simulink model "Ond_MLI_1"  (R2020a)
settings: Solver=VariableStepAuto  StartTime=0.0  StopTime=1  FixedStep=0.0001  RelTol=1e-3  EnableMultiTasking=on
InitFcn:
  | E=150;
  | V=220;
  | fs=50;
  | A=1;
  | 
  | Teta_0=0;
  | Cr=0;
  | Rr=3.805;
  | J=0.031;
  | f=0;
  | p=2;
  | Rs=4.85;
  | M=0.258;
  | Ls=0.274;
  | Lr=0.274;
  | R=[Rs 0 0 0;0 Rs 0 0;0 0 Rs 0;0 0 0 Rs];
  | L=[Ls 0 M 0;0 Ls 0 M;M 0 Lr 0;0 M 0 Lr];
  | A1=[0 -Ls 0 -M;Ls 0 M 0;0 0 0 0;0 0 0 0];
  | A2=[0 0 0 0;0 0 0 0;0 -M 0 -Lr;M 0 Lr 0];
undefined symbols (not defined in the file or in its folder): Vp
libraries: powerlib x21, simulink x2, powerlib_meascontrol x2
settings Model: SimulationMode=accelerator  Creator=SINA  LastModifiedBy=ABO-CHIFA
settings DataIOCC: ReturnWorkspaceOutputs=off
settings OptimizationCC: LifeSpan=inf
settings DebuggingCC: SFUnexpectedBacktrackingDiag=warning  SFNoUnconditionalDefaultTransitionDiag=warning  ArithmeticOperatorsInVariantConditions=warning
settings SFSimCC: SimUseLocalCustomCode=off  CustomCodeUndefinedFunction=UseInterfaceOnly
settings RTWCC: RTWUseLocalCustomCode=off
settings CodeAppCC: StateflowObjectComments=on
settings GRTTargetCC: TargetLangStandard=C89/C90 (ANSI)
settings ConfigComp: CovMetricSettings=dw  CovHtmlReporting=on  CovSaveCumulativeToWorkspaceVar=on  CovSaveSingleToWorkspaceVar=on  CovExternalEMLEnable=off
settings SimscapeCC: SimscapeNormalizeSystem=off

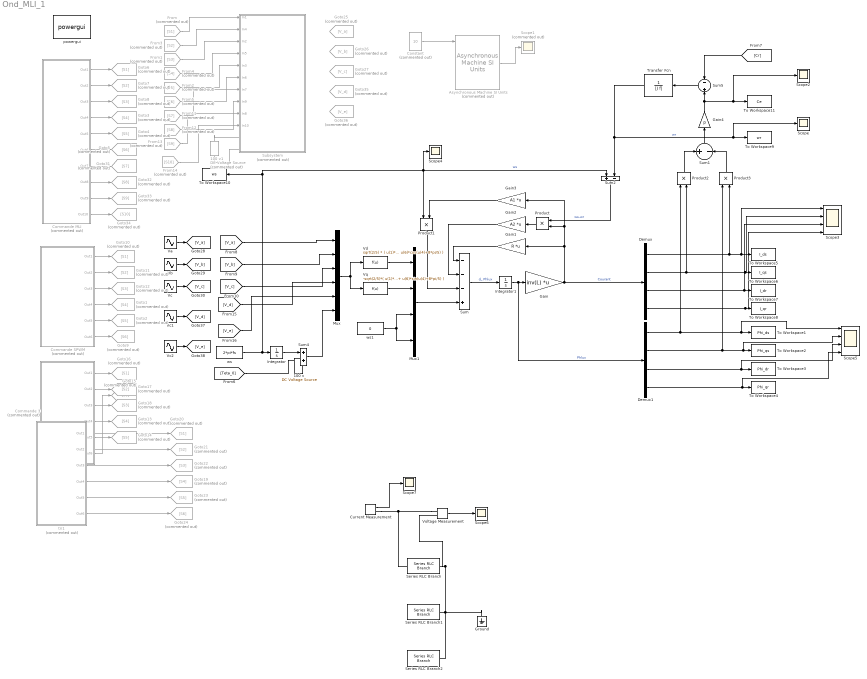
== system Ond_MLI_1 ==
  100 v : powerlib/Electrical Sources/DC Voltage Source  Amplitude=E  Measurements=Voltage
  100 v1 : powerlib/Electrical Sources/DC Voltage Source  Commented=on  Amplitude=E  Measurements=Voltage
  Asynchronous Machine SI Units : powerlib/Machines/Asynchronous Machine SI Units  Commented=on  RotorType=Squirrel-cage  PresetModel="15:  5.4 HP (4KW)   400 V  50Hz 1430 RPM"  MechanicalLoad=Torque Tm  ShowDetailedParameters=on  ReferenceFrame=Rotor  Units=SI  MeasurementBus=off  NominalParameters=[4000 400 50]  Stator=[1.405 0.005839]  Rotor=[1.395 0.005839]  Cage1=[0.4155 0.002066]  Cage2=[0.4168 0.0003495]  Lm=0.1722  Mechanical=[0.0131 0.002985 2]  PolePairs=2  InitialConditions=[1 0 0 0 0 0 0 0]  SimulateSaturation=off  Saturation=[14.03593122, 27.81365428, 53.79336849, 72.68890987, 97.98006896, 148.6815601, 215.7428561, 302.9841135, 428.7778367 ; 230, 322, 414, 460, 506, 552, 598, 644, 690]  LoadFlowParameters=1492000  TsPowergui=0  TsBlock=-1  IterativeModel=Trapezoidal non iterative  IterativeDiscreteModel=Trapezoidal non iterative  Pmec=1.492e+006
  "Commande 3 " : Subsystem  Commented=on
  "Commande MLI " : Subsystem  Commented=on
  "Commande SPWM " : Subsystem  Commented=on
  Constant : Constant  Commented=on  Value=10
  Current Measurement : powerlib/Measurements/Current Measurement  PhasorSimulation=off  OutputType=Complex  PSBequivalent=0
  Demux : Demux
  Demux1 : Demux
  From : From  Commented=on  GotoTag=S1
  From1 : From  Commented=on  GotoTag=S3
  From11 : From  Commented=on  GotoTag=S7
  From12 : From  Commented=on  GotoTag=S8
  From13 : From  Commented=on  GotoTag=S9
  From14 : From  Commented=on  GotoTag=S10
  From2 : From  Commented=on  GotoTag=S5
  From3 : From  Commented=on  GotoTag=S2
  From4 : From  Commented=on  GotoTag=S4
  From5 : From  Commented=on  GotoTag=S6
  Gain : Gain  Gain=inv(L)  Multiplication=Matrix(K*u)
  Gain1 : Gain  Gain=R  Multiplication=Matrix(K*u)
  Gain2 : Gain  Gain=A2  Multiplication=Matrix(K*u)
  Gain3 : Gain  Gain=A1  Multiplication=Matrix(K*u)
  Gain4 : Gain  Gain=p
  Goto{1,3,13,19} (4 alike) : Goto  Commented=on  GotoTag=S4
  Goto{6,10,16,20} (4 alike) : Goto  Commented=on  GotoTag=S1
  Goto{7,11,17,21} (4 alike) : Goto  Commented=on  GotoTag=S2
  Goto{8,12,18,22} (4 alike) : Goto  Commented=on  GotoTag=S3
  Goto{2,4,14,23} (4 alike) : Goto  Commented=on  GotoTag=S5
  Goto{5,9,15,24} (4 alike) : Goto  Commented=on  GotoTag=S6
  Goto25 : Goto  Commented=on  GotoTag=V_a
  Goto26 : Goto  Commented=on  GotoTag=V_b
  Goto27 : Goto  Commented=on  GotoTag=V_c
  Goto31 : Goto  Commented=on  GotoTag=S7
  Goto32 : Goto  Commented=on  GotoTag=S8
  Goto33 : Goto  Commented=on  GotoTag=S9
  Goto34 : Goto  Commented=on  GotoTag=S10
  Goto35 : Goto  Commented=on  GotoTag=V_d
  Goto36 : Goto  Commented=on  GotoTag=V_e
  Ground : powerlib/Elements/Ground  LConnTagsString=a
  Integrator : Integrator
  Integrator1 : Integrator
  Mux : Mux  Inputs=6
  Mux1 : Mux
  Product{,1..3} (4 alike) : Product
  Scope{,2,4,6..7} (5 alike) : Scope
  Scope1 : Scope  Commented=on
  Scope3 : Scope  NumInputPorts=4
  Scope5 : Scope  NumInputPorts=4
  Series RLC Branch : powerlib/Elements/Series RLC Branch  LConnTagsString=__new0  RConnTagsString=__new0  BranchType=R  Resistance=0.1  Inductance=1e-3  SetiL0=off  InitialCurrent=0  Capacitance=1e-6  Setx0=off  InitialVoltage=0  Measurements=None
  Series RLC Branch1 : powerlib/Elements/Series RLC Branch  LConnTagsString=__new0  RConnTagsString=__new0  BranchType=R  Resistance=0.1  Inductance=1e-3  SetiL0=off  InitialCurrent=0  Capacitance=1e-6  Setx0=off  InitialVoltage=0  Measurements=None
  Series RLC Branch2 : powerlib/Elements/Series RLC Branch  LConnTagsString=__new0  RConnTagsString=__new0  BranchType=R  Resistance=0.1  Inductance=1e-3  SetiL0=off  InitialCurrent=0  Capacitance=1e-6  Setx0=off  InitialVoltage=0  Measurements=None
  Subsystem : Subsystem  Commented=on
  Sum : Sum  Inputs=---+
  Sum1 : Sum  Inputs=+-
  Sum2 : Sum  Inputs=+-
  Sum4 : Sum
  Sum5 : Sum  Inputs=-+
  To Workspace1 : ToWorkspace  VariableName=Phi_ds  SampleTime=-1
  To Workspace10 : ToWorkspace  VariableName=ws  SampleTime=-1
  To Workspace11 : ToWorkspace  VariableName=Ce  SampleTime=-1
  To Workspace2 : ToWorkspace  VariableName=Phi_qs  SampleTime=-1
  To Workspace3 : ToWorkspace  VariableName=Phi_dr  SampleTime=-1
  To Workspace4 : ToWorkspace  VariableName=Phi_qr  SampleTime=-1
  To Workspace5 : ToWorkspace  VariableName=I_ds  SampleTime=-1
  To Workspace6 : ToWorkspace  VariableName=I_qs  SampleTime=-1
  To Workspace7 : ToWorkspace  VariableName=I_dr  SampleTime=-1
  To Workspace8 : ToWorkspace  VariableName=I_qr  SampleTime=-1
  To Workspace9 : ToWorkspace  VariableName=wr  SampleTime=-1
  Transfer Fcn : TransferFcn  Denominator=[J f]
  Va : Sin  Amplitude=V*sqrt(2)  Frequency=2*pi*fs  SampleTime=0
  Vb : Sin  Amplitude=V*sqrt(2)  Frequency=2*pi*fs  Phase=2*pi/5  SampleTime=0
  Vc : Sin  Amplitude=V*sqrt(2)  Frequency=2*pi*fs  Phase=4*pi/5  SampleTime=0
  Vc1 : Sin  Amplitude=V*sqrt(2)  Frequency=2*pi*fs  Phase=6*pi/5  SampleTime=0
  Vc2 : Sin  Amplitude=V*sqrt(2)  Frequency=2*pi*fs  Phase=8*pi/5  SampleTime=0
  Vd : Fcn  Expr="sqrt(2/5) * ( u(1)*cos(u(4))  + u(2)*cos(u(4)+2*pi/5) + u(3)*cos(u(4)+4*pi/5)+ u(5)*cos(u(4)+6*pi/5)+ u(6)*cos(u(4)+8*pi/5) )"
  Voltage Measurement : powerlib/Measurements/Voltage Measurement  PhasorSimulation=off  OutputType=Complex  PSBequivalent=0
  Vq : Fcn  Expr="-sqrt(2/5)*( u(1)*sin(u(4))  + u(2)*sin(u(4)+2*pi/5) + u(3)*sin(u(4)+4*pi/5)+ u(5)*sin(u(4)+6*pi/5)+ u(6)*sin(u(4)+8*pi/5) )"
  powergui : powerlib/powergui  Priority=1  SimulationMode=Discrete  SampleTime=1e-6  frequency=60  Iterations=50  frequencyindice=0  Pbase=100e6  ErrMax=1e-4  UnitsV=kV  UnitsW=MW  buscounter=0  FunctionMessages=off  echomessages=off  EnableUseOfTLC=off  CurrentSourceSwitches=off  DisableSnubberDevices=off  DisableRonSwitches=off  DisableVfSwitches=off  DisplayEquations=off  AutomaticDiscreteSolvers=off  SolverType=Tustin/Backward Euler (TBE)  Interpol=off  ExternalGateDelay=off  methode=off  Ts=10  x0status=blocks  SPID=off  SwTol=0  HookPort=off  NonlinearTolerance=1e-4  nMaxIteration=100  ContinueOnMaxIteration=off  RestoreLinks=warning  ResistiveCurrentMeasurement=off  Frange=[0:2:500]  Ylog=off  Xlog=on  ShowGrid=off  save=off  variable=ZData  structure=0  ZoomFFT=off  StartTime=0.0  cycles=1  DisplayStyle=1  fundamental=60  FreqAxis=off  MaxFrequency=1000  frequencyindicesteady=1  RmsSteady=1  display=off
  "tri1 " : Subsystem  Commented=on
  ws : Constant  Value=2*pi*fs
  ws1 : Constant  Value=0
  wires:
  "Commande MLI "/4(Out4) -> Goto3/1
  "Commande MLI "/5(Out5) -> Goto4/1
  "Commande MLI "/6(Out6) -> Goto5/1
  "Commande MLI "/2(Out2) -> Goto7/1
  "Commande MLI "/1(Out1) -> Goto6/1
  "Commande MLI "/3(Out3) -> Goto8/1
  "Commande SPWM "/1(Out1) -> Goto10/1
  "Commande SPWM "/2(Out2) -> Goto11/1
  "Commande SPWM "/3(Out3) -> Goto12/1
  "Commande SPWM "/4(Out4) -> Goto1/1
  "Commande SPWM "/5(Out5) -> Goto2/1
  "Commande SPWM "/6(Out6) -> Goto9/1
  From/1 -> Subsystem/1(In1)
  From1/1 -> Subsystem/3(In2)
  From2/1 -> Subsystem/5(In3)
  From3/1 -> Subsystem/2(In4)
  From4/1 -> Subsystem/4(In5)
  From5/1 -> Subsystem/6(In6)
  "Commande 3 "/1(Out1) -> Goto16/1
  "Commande 3 "/2(Out2) -> Goto17/1
  "Commande 3 "/3(Out3) -> Goto18/1
  "Commande 3 "/4(Out4) -> Goto13/1
  "Commande 3 "/5(Out5) -> Goto14/1
  "Commande 3 "/6(Out6) -> Goto15/1
  Asynchronous Machine SI Units/1 -> Scope1/1
  Constant/1 -> Asynchronous Machine SI Units/1
  "tri1 "/1(Out1) -> Goto20/1
  "tri1 "/2(Out2) -> Goto21/1
  "tri1 "/3(Out3) -> Goto22/1
  "tri1 "/4(Out4) -> Goto19/1
  "tri1 "/5(Out5) -> Goto23/1
  "tri1 "/6(Out6) -> Goto24/1
  ws/1 -> Sum2/1, Scope4/1, Product1/1, To Workspace10/1, Integrator/1  "ws"
  Mux/1 -> Vd/1, Vq/1
  Vd/1 -> Mux1/1
  Vq/1 -> Mux1/2
  ws1/1 -> Mux1/3, Mux1/4
  Sum/1 -> Integrator1/1  "d_ Phlux"
  Integrator1/1 -> Gain/1, Demux1/1  "Phlux"
  Gain/1 -> Demux/1, Gain3/1, Product/2, Gain1/1  "Courant"
  Product/1 -> Gain2/1
  Gain3/1 -> Product1/2
  Demux1/1 -> Product2/1, Scope5/1, To Workspace1/1
  Demux1/4 -> Scope5/4, To Workspace4/1
  Demux1/3 -> Scope5/3, To Workspace3/1
  Demux/4 -> Scope3/4, To Workspace8/1
  Demux/3 -> Scope3/3, To Workspace7/1
  Demux/2 -> Scope3/2, To Workspace6/1, Product2/2
  Demux/1 -> Scope3/1, To Workspace5/1, Product3/2
  Demux1/2 -> Product3/1, Scope5/2, To Workspace2/1
  Product2/1 -> Sum1/1
  Product3/1 -> Sum1/2
  Transfer Fcn/1 -> To Workspace9/1, Scope/1, Sum2/2  "wr"
  Sum2/1 -> Product/1  "ws-wr"
  Sum1/1 -> Gain4/1
  Integrator/1 -> Sum4/1
  [Teta_0] -> Sum4/2
  Sum5/1 -> Transfer Fcn/1
  Gain4/1 -> Sum5/2, To Workspace11/1, Scope2/1
  [V_a] -> Mux/1
  [V_b] -> Mux/2
  Vb/1 -> [V_b]
  Va/1 -> [V_a]
  Vc/1 -> [V_c]
  [V_c] -> Mux/3
  Mux1/1 -> Sum/4
  Product1/1 -> Sum/3
  Gain2/1 -> Sum/2
  Gain1/1 -> Sum/1
  [Cr] -> Sum5/1
  "Commande MLI "/7(Out7) -> Goto31/1
  "Commande MLI "/8(Out8) -> Goto32/1
  "Commande MLI "/9(Out9) -> Goto33/1
  "Commande MLI "/10(Out10) -> Goto34/1
  From11/1 -> Subsystem/7(In7)
  From12/1 -> Subsystem/8(In9)
  From13/1 -> Subsystem/9(In8)
  From14/1 -> Subsystem/10(In10)
  Sum4/1 -> Mux/6
  [V_d] -> Mux/4
  [V_e] -> Mux/5
  Vc1/1 -> [V_d]
  Vc2/1 -> [V_e]
  Current Measurement/1 -> Scope7/1
  Voltage Measurement/1 -> Scope6/1
  connections:
  100 v1/RConn1 -- Subsystem/LConn1
  100 v1/LConn1 -- Subsystem/LConn2
  Series RLC Branch1/RConn1 -- Ground/LConn1 -- Series RLC Branch2/RConn1 -- Series RLC Branch/RConn1 -- Voltage Measurement/LConn2
  Voltage Measurement/LConn1 -- Current Measurement/RConn1 -- Series RLC Branch/LConn1

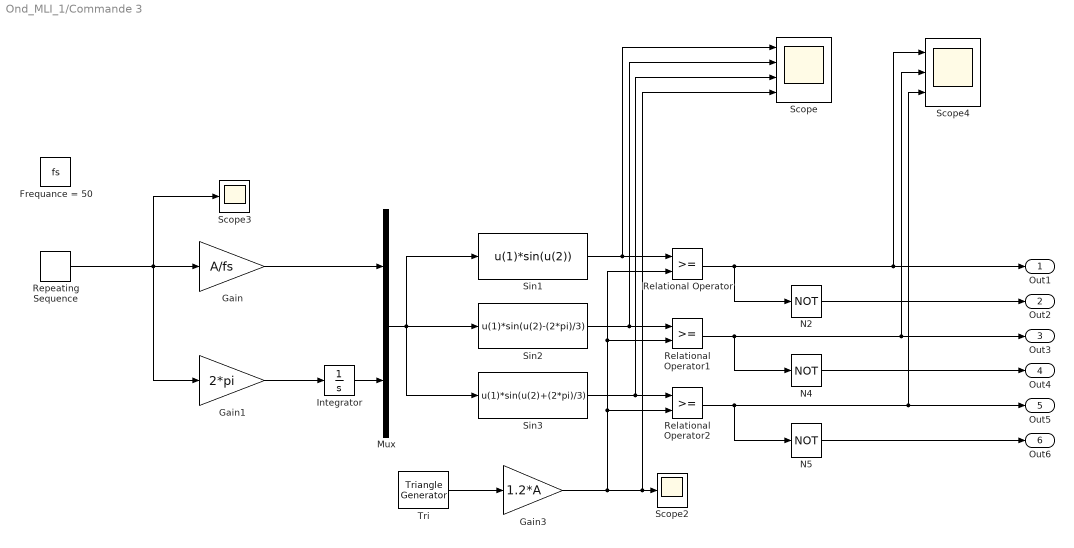
== system Ond_MLI_1/Commande 3  ==
  Frequance = 50 : Constant  Value=fs
  Gain : Gain  Gain=A/fs
  Gain1 : Gain  Gain=2*pi
  Gain3 : Gain  Gain=1.2*A
  Integrator : Integrator
  Mux : Mux  Inputs=2
  N2 : Logic  Operator=NOT  AllPortsSameDT=off  OutDataTypeStr=boolean
  N4 : Logic  Operator=NOT  AllPortsSameDT=off  OutDataTypeStr=boolean
  N5 : Logic  Operator=NOT  AllPortsSameDT=off  OutDataTypeStr=boolean
  Relational Operator : RelationalOperator  OutDataTypeStr=boolean  RndMeth=Nearest
  Relational Operator1 : RelationalOperator  OutDataTypeStr=boolean  RndMeth=Nearest
  Relational Operator2 : RelationalOperator  OutDataTypeStr=boolean  RndMeth=Nearest
  Repeating Sequence : simulink/Sources/Repeating Sequence  rep_seq_t=[0 0.1 10]  rep_seq_y=[0 fs fs]
  Scope : Scope  NumInputPorts=4
  Scope2 : Scope
  Scope3 : Scope
  Scope4 : Scope  NumInputPorts=3
  Sin1 : Fcn  Expr=u(1)*sin(u(2))
  Sin2 : Fcn  Expr=u(1)*sin(u(2)-(2*pi)/3)
  Sin3 : Fcn  Expr=u(1)*sin(u(2)+(2*pi)/3)
  Tri : powerlib_meascontrol/Pulse & Signal Generators/Triangle Generator  Freq=1e3  Phase=90  Ts=0
  Out1 : Outport
  Out2 : Outport  Port=2
  Out3 : Outport  Port=3
  Out4 : Outport  Port=4
  Out5 : Outport  Port=5
  Out6 : Outport  Port=6
  wires:
  Gain1/1 -> Integrator/1
  Integrator/1 -> Mux/2
  Gain/1 -> Mux/1
  Mux/1 -> Sin3/1, Sin2/1, Sin1/1
  N2/1 -> Out2/1
  N4/1 -> Out4/1
  Relational Operator2/1 -> N5/1, Out5/1, Scope4/3
  Gain3/1 -> Relational Operator2/2, Relational Operator1/2, Relational Operator/2, Scope2/1, Scope/4
  Tri/1 -> Gain3/1
  Sin1/1 -> Relational Operator/1, Scope/1
  Sin2/1 -> Relational Operator1/1, Scope/2
  Sin3/1 -> Relational Operator2/1, Scope/3
  N5/1 -> Out6/1
  Relational Operator1/1 -> N4/1, Out3/1, Scope4/2
  Relational Operator/1 -> Out1/1, Scope4/1, N2/1
  Repeating Sequence/1 -> Gain1/1, Scope3/1, Gain/1

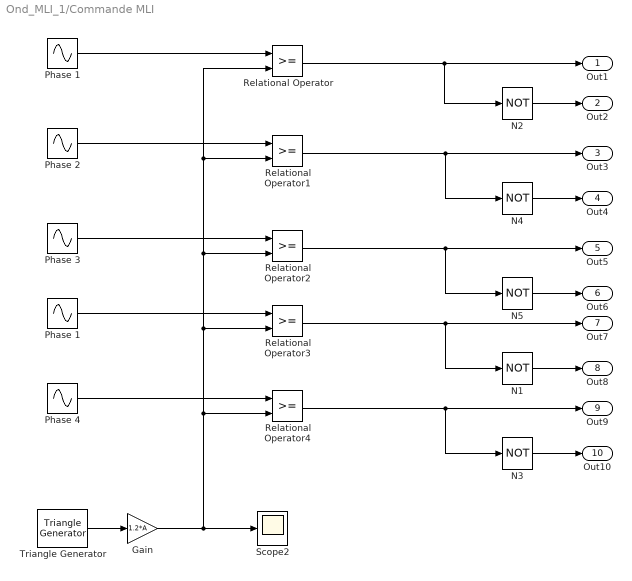
== system Ond_MLI_1/Commande MLI  ==
  Gain : Gain  Gain=1.2*A
  N{1..5} (5 alike) : Logic  Operator=NOT  AllPortsSameDT=off  OutDataTypeStr=boolean
  Phase 1 : Sin  Amplitude=A  Frequency=2*pi*fs  Phase=6*pi/5  SampleTime=0
  "Phase 1 " : Sin  Amplitude=A  Frequency=2*pi*fs  SampleTime=0
  Phase 2 : Sin  Amplitude=A  Frequency=2*pi*fs  Phase=2*pi/5  SampleTime=0
  Phase 3 : Sin  Amplitude=A  Frequency=2*pi*fs  Phase=4*pi/5  SampleTime=0
  Phase 4 : Sin  Amplitude=A  Frequency=2*pi*fs  Phase=8*pi/5  SampleTime=0
  Relational Operator{,1..4} (5 alike) : RelationalOperator  OutDataTypeStr=boolean  RndMeth=Nearest
  Scope2 : Scope
  Triangle Generator : powerlib_meascontrol/Pulse & Signal Generators/Triangle Generator  Freq=1e3  Phase=90  Ts=0
  Out1 : Outport
  Out2 : Outport  Port=2
  Out3 : Outport  Port=3
  Out4 : Outport  Port=4
  Out5 : Outport  Port=5
  Out6 : Outport  Port=6
  Out7 : Outport  Port=7
  Out8 : Outport  Port=8
  Out9 : Outport  Port=9
  Out10 : Outport  Port=10
  wires:
  Phase 3/1 -> Relational Operator2/1
  N4/1 -> Out4/1
  N5/1 -> Out6/1
  N2/1 -> Out2/1
  Relational Operator/1 -> N2/1, Out1/1
  Relational Operator1/1 -> Out3/1, N4/1
  Relational Operator2/1 -> Out5/1, N5/1
  Phase 2/1 -> Relational Operator1/1
  "Phase 1 "/1 -> Relational Operator/1
  Triangle Generator/1 -> Gain/1
  Gain/1 -> Relational Operator4/2, Relational Operator3/2, Relational Operator2/2, Relational Operator1/2, Relational Operator/2, Scope2/1
  Relational Operator3/1 -> Out7/1, N1/1
  N1/1 -> Out8/1
  Phase 1/1 -> Relational Operator3/1
  Phase 4/1 -> Relational Operator4/1
  N3/1 -> Out10/1
  Relational Operator4/1 -> Out9/1, N3/1

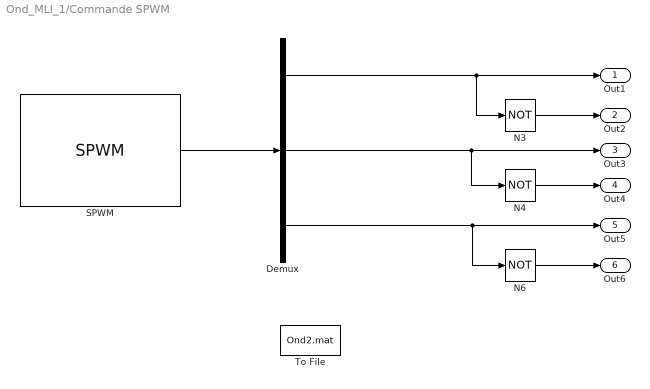
== system Ond_MLI_1/Commande SPWM  ==
  Demux : Demux  Outputs=3
  N3 : Logic  Operator=NOT  AllPortsSameDT=off  OutDataTypeStr=boolean
  N4 : Logic  Operator=NOT  AllPortsSameDT=off  OutDataTypeStr=boolean
  N6 : Logic  Operator=NOT  AllPortsSameDT=off  OutDataTypeStr=boolean
  SPWM : S-Function  FunctionName=SPWM  Parameters=""  SFunctionDeploymentMode=off  EnableBusSupport=off
  To File : ToFile  Filename=Ond2.mat  SaveFormat=Timeseries
  Out1 : Outport
  Out2 : Outport  Port=2
  Out3 : Outport  Port=3
  Out4 : Outport  Port=4
  Out5 : Outport  Port=5
  Out6 : Outport  Port=6
  wires:
  Demux/2 -> Out3/1, N4/1
  N4/1 -> Out4/1
  Demux/1 -> Out1/1, N3/1
  N6/1 -> Out6/1
  N3/1 -> Out2/1
  Demux/3 -> Out5/1, N6/1
  SPWM/1 -> Demux/1

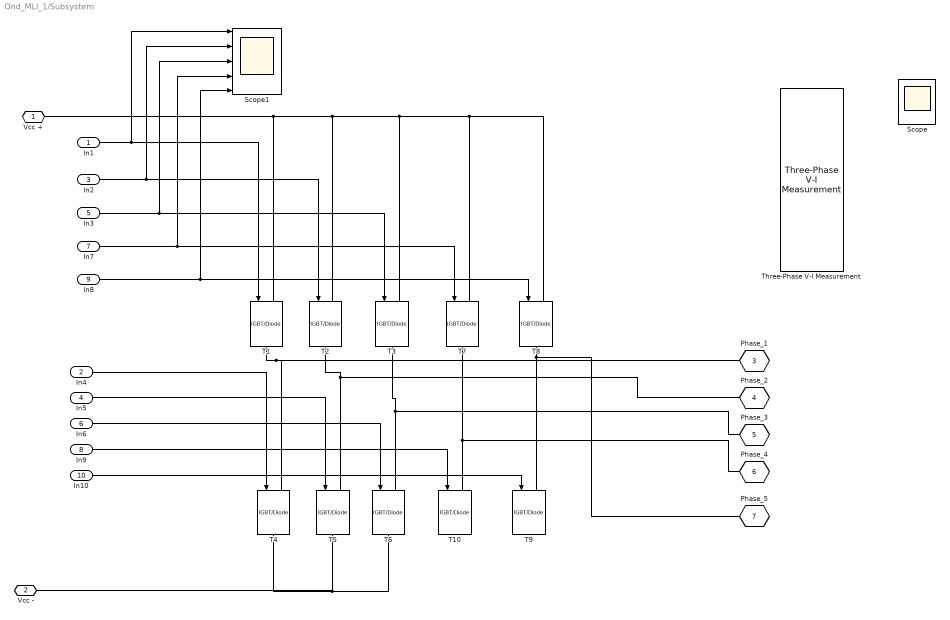
== system Ond_MLI_1/Subsystem ==
  In1 : Inport
  In4 : Inport  Port=2
  In2 : Inport  Port=3
  In5 : Inport  Port=4
  In3 : Inport  Port=5
  In6 : Inport  Port=6
  In7 : Inport  Port=7
  In9 : Inport  Port=8
  In8 : Inport  Port=9
  In10 : Inport  Port=10
  Scope : Scope  NumInputPorts=2
  Scope1 : Scope  NumInputPorts=5
  T{1..10} (10 alike) : powerlib/Power Electronics/IGBT//Diode  Ron=1e-3  Rs=1e5  Cs=inf  Measurements=off
  Three-Phase V-I Measurement : powerlib/Measurements/Three-Phase V-I Measurement  VoltageMeasurement=phase-to-ground  SetLabelV=off  LabelV=Vabc  Vpu=off  VpuLL=off  CurrentMeasurement=yes  SetLabelI=off  LabelI=Iabc  Ipu=off  Pbase=100e6  Vbase=500e3  OutputType=Complex  PhasorSimulation=off  PSBequivalent=0
  Vcc + : PMIOPort  Side=Left
  Vcc - : PMIOPort  Port=2  Side=Left
  Phase_1 : PMIOPort  Tag=PMCPort  Port=3  Side=Right
  Phase_2 : PMIOPort  Tag=PMCPort  Port=4  Side=Right
  Phase_3 : PMIOPort  Tag=PMCPort  Port=5  Side=Right
  Phase_4 : PMIOPort  Tag=PMCPort  Port=6  Side=Right
  Phase_5 : PMIOPort  Tag=PMCPort  Port=7  Side=Right
  wires:
  In1/1 -> Scope1/1, T1/1
  In2/1 -> Scope1/2, T2/1
  In3/1 -> Scope1/3, T3/1
  In7/1 -> Scope1/4, T7/1
  In8/1 -> Scope1/5, T8/1
  In4/1 -> T4/1
  In5/1 -> T5/1
  In6/1 -> T6/1
  In9/1 -> T10/1
  In10/1 -> T9/1
  connections:
  T5/RConn1 -- T4/RConn1 -- Vcc -/RConn1 -- T6/RConn1
  Vcc +/RConn1 -- T1/LConn1 -- T2/LConn1 -- T3/LConn1 -- T8/LConn1 -- T7/LConn1
  T9/LConn1 -- Phase_5/RConn1 -- T8/RConn1
  T10/LConn1 -- T7/RConn1 -- Phase_4/RConn1
  T6/LConn1 -- Phase_3/RConn1 -- T3/RConn1
  T5/LConn1 -- Phase_2/RConn1 -- T2/RConn1
  T4/LConn1 -- Phase_1/RConn1 -- T1/RConn1

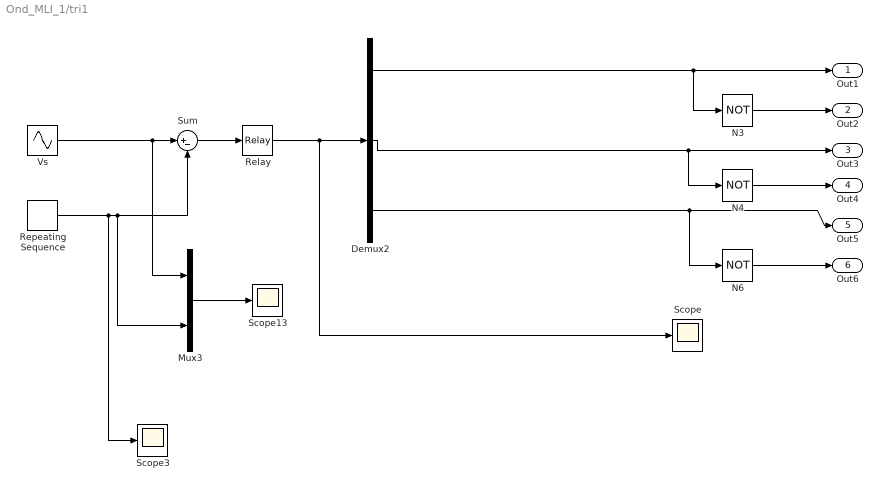
== system Ond_MLI_1/tri1  ==
  Demux2 : Demux  Outputs=3
  Mux3 : Mux  Inputs=2
  N3 : Logic  Operator=NOT  AllPortsSameDT=off  OutDataTypeStr=boolean
  N4 : Logic  Operator=NOT  AllPortsSameDT=off  OutDataTypeStr=boolean
  N6 : Logic  Operator=NOT  AllPortsSameDT=off  OutDataTypeStr=boolean
  Relay : Relay
  Repeating Sequence : simulink/Sources/Repeating Sequence  rep_seq_t="[0 1  2]/5000"  rep_seq_y=[-Vp Vp -Vp]
  Scope : Scope
  Scope13 : Scope
  Scope3 : Scope
  Sum : Sum  Inputs=|+-
  Vs : Sin  Amplitude=A  Frequency=2*pi*fs  Phase=[0 -2*pi/3 2*pi/3]  SampleTime=0
  Out1 : Outport
  Out2 : Outport  Port=2
  Out3 : Outport  Port=3
  Out4 : Outport  Port=4
  Out5 : Outport  Port=5
  Out6 : Outport  Port=6
  wires:
  Vs/1 -> Sum/1, Mux3/1
  Repeating Sequence/1 -> Scope3/1, Sum/2, Mux3/2
  Sum/1 -> Relay/1
  Mux3/1 -> Scope13/1
  N3/1 -> Out2/1
  Demux2/3 -> N6/1, Out5/1
  Demux2/1 -> N3/1, Out1/1
  N4/1 -> Out4/1
  N6/1 -> Out6/1
  Relay/1 -> Scope/1, Demux2/1
  Demux2/2 -> Out3/1, N4/1
